simulink model "dummyModel"  (R2021a)
settings: Solver=FixedStepDiscrete  StartTime=0.0  StopTime=inf  RelTol=1e-3
libraries: simulink x1, sysauto_lib x1
settings Model: RequirementInfo="{}  %GIDa_9af0a4cd_5f44_4d95_97ed_12e2ef6ba56d"  Creator=mhochstrasser  LastModifiedBy=ge46fox
settings SolverCC: AlgebraicLoopSolver=TrustRegion  AutoInsertRateTranBlk=on
settings DataIOCC: LimitDataPoints=on  SaveOutput=off  SignalLogging=off  DSMLogging=off  SaveTime=off  ReturnWorkspaceOutputs=off
settings OptimizationCC: LifeSpan=inf
settings DebuggingCC: AlgebraicLoopMsg=error  SingleTaskRateTransMsg=error  AllowSymbolicDim=off  SFUnexpectedBacktrackingDiag=warning  SFNoUnconditionalDefaultTransitionDiag=warning  SFExecutionAtInitializationDiag=none  SFMachineParentedDataDiag=warning  ArithmeticOperatorsInVariantConditions=warning
settings SFSimCC: SimUseLocalCustomCode=off  CustomCodeUndefinedFunction=UseInterfaceOnly
settings RTWCC: RTWUseLocalCustomCode=off
settings CodeAppCC: StateflowObjectComments=on
settings GRTTargetCC: TargetLangStandard=C89/C90 (ANSI)

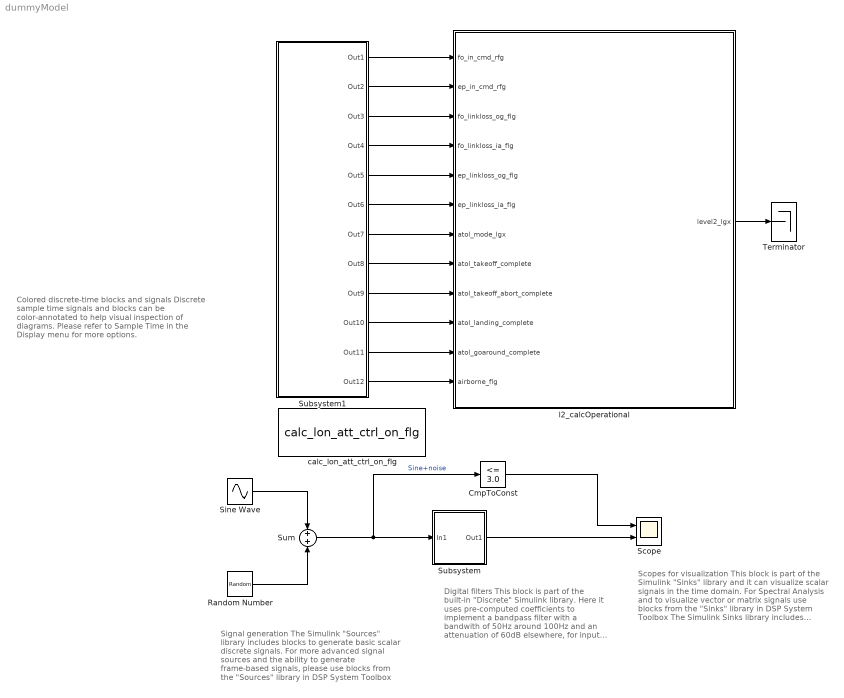
== system dummyModel ==
  note: Signal generation
      | The Simulink "Sources" library includes blocks to generate basic scalar discrete signals.
      | For more advanced signal sources and the ability to generate frame-based signals, please use blocks from the "Sources" library in DSP System Toolbox
  note: Scopes for visualization
      | This block is part of the Simulink "Sinks" library and it can visualize scalar signals in the time domain.
      | For Spectral Analysis and to visualize vector or matrix signals use blocks from the "Sinks" library in DSP System Toolbox
      |
      | The Simulink Sinks library includes scopes to visualize scalar signals in the time domain. For the Spectrum Analyzer and to viasualize vector or matrix signals refer to the Sinks library of DSP System Toolbox
  note: Digital filters
      | This block is part of the built-in "Discrete" Simulink library. Here it uses pre-computed coefficients to implement a bandpass filter with a bandwith of 50Hz around 100Hz and an attenuation of 60dB elsewhere, for input signals sampled at 8kHz.
      | To design digital filters, to select specific implementation structures, or to simulate fixed-point arithmetic use blocks from the "Filtering" library in DSP System Toolbox
  note: Colored discrete-time blocks and signals
      | Discrete sample time signals and blocks can be color-annotated to help visual inspection of diagrams. Please refer to Sample Time in the Display menu for more options.
  CmpToConst : simulink/Logic and Bit Operations/Compare To Constant  relop=<=  const=3.0  OutDataTypeStr=boolean
  Random Number : RandomNumber  RequirementInfo="{}  %GIDa_aef719ec_22fa_4968_b9f2_caf883574260"  SampleTime=1/8000
  Scope : Scope  NumInputPorts=2
  Sine Wave : Sin  Frequency=2*pi*100  Samples=1  SampleTime=1/8000
  Subsystem : Subsystem
  Subsystem1 : Subsystem
  Sum : Sum
  Terminator : Terminator
  calc_lon_att_ctrl_on_flg : sysauto_lib/calc_lon_att_ctrl_on_flg  SystemSampleTime=-1  VariantActivationTime=update diagram  Latency=0  AutoFrameSizeCalculation=off
  l2_calcOperational : Stateflow chart  TreatAsAtomicUnit=on
      settings: RTWSystemCode=Inline
  wires:
  Sum/1 -> CmpToConst/1, Subsystem/1(In1)  "Sine+noise"
  Sine Wave/1 -> Sum/1
  Random Number/1 -> Sum/2
  Subsystem/1(Out1) -> Scope/2
  CmpToConst/1 -> Scope/1
  l2_calcOperational/1(level2_lgx) -> Terminator/1
  Subsystem1/1(Out1) -> l2_calcOperational/1(fo_in_cmd_rfg)
  Subsystem1/2(Out2) -> l2_calcOperational/2(ep_in_cmd_rfg)
  Subsystem1/3(Out3) -> l2_calcOperational/3(fo_linkloss_og_flg)
  Subsystem1/4(Out4) -> l2_calcOperational/4(fo_linkloss_ia_flg)
  Subsystem1/5(Out5) -> l2_calcOperational/5(ep_linkloss_og_flg)
  Subsystem1/6(Out6) -> l2_calcOperational/6(ep_linkloss_ia_flg)
  Subsystem1/7(Out7) -> l2_calcOperational/7(atol_mode_lgx)
  Subsystem1/8(Out8) -> l2_calcOperational/8(atol_takeoff_complete)
  Subsystem1/9(Out9) -> l2_calcOperational/9(atol_takeoff_abort_complete)
  Subsystem1/10(Out10) -> l2_calcOperational/10(atol_landing_complete)
  Subsystem1/11(Out11) -> l2_calcOperational/11(atol_goaround_complete)
  Subsystem1/12(Out12) -> l2_calcOperational/12(airborne_flg)

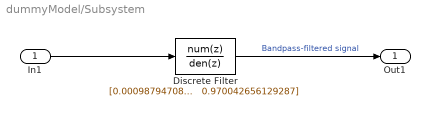
== system dummyModel/Subsystem ==
  In1 : Inport
  Discrete Filter : DiscreteFilter  RequirementInfo="{}  %GIDa_1e970cd2_fa55_4b33_ada7_a6ab44b2a5d3"  Numerator="[0.000987947087024  -0.007866111001516   0.027438142026555  -0.054764720946282   0.068409485670105  -0.054764720946282   0.027438142026555  -0.007866111001516   0.000987947087024]"  Denominator="[1.000000000000000  -7.944031997545686  27.635065757644615 -54.984635962907035  68.438574736652072 -54.568127619544200  27.217980746836638  -7.764868315600190   0.970042656129287]"
  Out1 : Outport
  wires:
  In1/1 -> Discrete Filter/1
  Discrete Filter/1 -> Out1/1  "Bandpass-filtered signal"

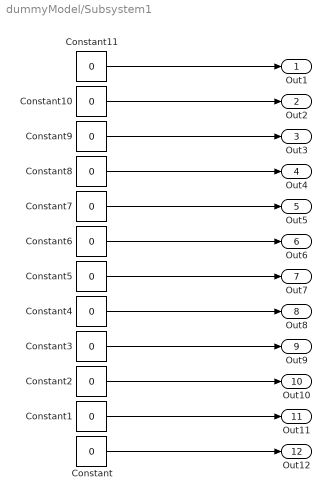
== system dummyModel/Subsystem1 ==
  Constant{,1..11} (12 alike) : Constant  Value=0  OutDataTypeStr=Inherit: Inherit via back propagation
  Out1 : Outport
  Out2 : Outport  Port=2
  Out3 : Outport  Port=3
  Out4 : Outport  Port=4
  Out5 : Outport  Port=5
  Out6 : Outport  Port=6
  Out7 : Outport  Port=7
  Out8 : Outport  Port=8
  Out9 : Outport  Port=9
  Out10 : Outport  Port=10
  Out11 : Outport  Port=11
  Out12 : Outport  Port=12
  wires:
  Constant1/1 -> Out11/1
  Constant7/1 -> Out5/1
  Constant8/1 -> Out4/1
  Constant/1 -> Out12/1
  Constant5/1 -> Out7/1
  Constant11/1 -> Out1/1
  Constant3/1 -> Out9/1
  Constant6/1 -> Out6/1
  Constant9/1 -> Out3/1
  Constant10/1 -> Out2/1
  Constant2/1 -> Out10/1
  Constant4/1 -> Out8/1

== stateflow chart dummyModel/l2_calcOperational ==
  settings: stateMachineType=MEALY_MACHINE
  state fo_in_cmd
  state ep_in_cmd
  state ep_linkloss
  state tc [group]
    state result = foincmd_folinkloss [function]
      note: /*
          | Switch from EP to FCC if either ep_linkloss or interface_error,
          | but only if the aircraft is flying, therefore a special on ground
          | link loss behaviour can be implemented
          | */
      note: /*
          |     This function is true,
          |     when ATOL prohibts automatic transition to linkloss
          | */
      (default) -> (junction 293)
      (junction 293) -> (junction 309) [order 2]
      (junction 293) -> (junction 183) [order 1] : [(((fo_linkloss_ia_flg == true)&&(airborne_flg == true))||...
          | ((fo_linkloss_og_flg == true)&&(airborne_flg == false)))]
      (junction 309) -> (junction 305) : {result = false;}
      (junction 183) -> (junction 316) [order 1] : [((atol_mode_lgx == uint8(40))&&...
          | (atol_takeoff_complete == false))||...
          | ((atol_mode_lgx == uint8(41))&&...
          | (atol_takeoff_abort_complete == false))]
      (junction 183) -> (junction 297) [order 2]
      (junction 316) -> (junction 314) : {result = false;}
      (junction 297) -> (junction 317) [order 1] : [((atol_mode_lgx == uint8(42))&&...
          | (atol_landing_complete == false))||...
          | ((atol_mode_lgx == uint8(43))&&...
          | (atol_goaround_complete == false))]
      (junction 297) -> (junction 298) [order 2] : {result = true;}
      (junction 317) -> (junction 315) : {result = false;}
      (junction 315) -> (junction 298)
      (junction 314) -> (junction 315)
      (junction 305) -> (junction 314)
    state result = x_epincmd [function]
      note: // change to EP if rising edge is detected on ep_in_cmd
      (default) -> (junction 198)
      (junction 198) -> (junction 239) [order 1] : [ep_in_cmd_rfg == true]
      (junction 198) -> (junction 197) [order 2] : {result = false;}
      (junction 239) -> (junction 240) : {result = true;}
      (junction 197) -> (junction 240)
    state result = x_foincmd [function]
      note: // change to FO if rising edge is detected on fo_in_cmd,
          | //but only if no rising edge is detected for ep_in_cmd
          | // this is needed for state ep_in_cmd transition inhibit
          | //[hasChangedTo(fao_in_cmd_flg, 1) &~ (hasChangedTo(ep_in_cmd_flg, 1))]
      (default) -> (junction 252)
      (junction 252) -> (junction 251) [order 1] : [(fo_in_cmd_rfg == true)&&...
          | (ep_in_cmd_rfg == false)]
      (junction 252) -> (junction 253) [order 2] : {result = false;}
      (junction 251) -> (junction 255) : {result = true;}
      (junction 253) -> (junction 255)
    state result = epincmd_eplinkloss [function]
      note: /*
          | Switch from EP to FCC if either ep_linkloss or interface_error,
          | but only if the aircraft is flying, therefore a special on ground
          | link loss behaviour can be implemented
          | */
      (default) -> (junction 154) : [((ep_linkloss_ia_flg == true)&&(airborne_flg == true))||...
          | ((ep_linkloss_og_flg == true)&&(airborne_flg == false))]
      (junction 154) -> (junction 156) : {result = true;}
  state ta [group]
    state foincmd_folinkloss [function]
      (default) -> (junction 134) : {level2_lgx = 2;}
    state x_epincmd [function]
      (default) -> (junction 202) : {level2_lgx = 4;}
    state x_foincmd [function]
      (default) -> (junction 212) : {level2_lgx = 5;}
    state epincmd_eplinkloss [function]
      (default) -> (junction 143) : {level2_lgx = 3;}
  state fo_linkloss
  note: ATOL is not part of this statemachine because it would lead to either (ATOL can be exited any time by any other mode commanded by fo)
      | - a inconsitent behaiviour for the fo, example: atol with no gps, he wants hlc, hlc is not possible, therefore he gets mlc (standart mode), in all other modes if he commands one mode that isn't possible he stays in the current mode
      | - many TCs that are manly used within the fo_cmd statemachine, like mode cmds, availablity
      |
      | the second possibility makes more sense but than atol is like every other mode and is therefore not avaible here but within the fo_in_cmd statemaschine
  note: © TUM-FSD, Developer: C.Krause
  fo_in_cmd -> (junction 45) [order 1] : [tc.x_epincmd() == true]
  (junction 45) -> (junction 17)
  (junction 42) -> fo_in_cmd : {ta.x_foincmd()}
  (junction 20) -> (junction 42)
  (junction 256) -> fo_in_cmd : {ta.x_foincmd()}
  fo_in_cmd -> (junction 38) [order 2] : [tc.foincmd_folinkloss() == true]
  (junction 214) -> (junction 256) [order 2] : [tc.x_foincmd() == true]
  (junction 17) -> ep_in_cmd : {ta.x_epincmd()}
  (junction 81) -> (junction 17)
  ep_in_cmd -> (junction 20) [order 1] : [tc.x_foincmd() == true]
  (junction 86) -> (junction 20)
  (junction 258) -> ep_in_cmd : {ta.x_epincmd()}
  (default) -> (junction 214)
  (junction 214) -> (junction 258) [order 1] : [tc.x_epincmd() == true]
  (junction 214) -> (junction 231) [order 3]
  ep_in_cmd -> (junction 83) [order 2] : [tc.epincmd_eplinkloss() == true]
  ep_linkloss -> (junction 86) [order 2] : [tc.x_foincmd() == true]
  (junction 91) -> (junction 86)
  (junction 231) -> (junction 83)
  (junction 83) -> ep_linkloss : {ta.epincmd_eplinkloss()}
  ep_linkloss -> (junction 81) [order 1] : [tc.x_epincmd() == true]
  (junction 88) -> (junction 81)
  fo_linkloss -> (junction 91) [order 2] : [tc.x_foincmd() == true]
  (junction 38) -> fo_linkloss : {ta.foincmd_folinkloss()}
  fo_linkloss -> (junction 88) [order 1] : [tc.x_epincmd() == true]
  data: result function_output boolean; result function_output boolean; result function_output boolean; result function_output boolean; fo_in_cmd_rfg input boolean; ep_in_cmd_rfg input boolean; fo_linkloss_og_flg input boolean; fo_linkloss_ia_flg input boolean; ep_linkloss_og_flg input boolean; ep_linkloss_ia_flg input boolean; level2_lgx output int32; atol_mode_lgx input uint8; atol_takeoff_complete input boolean; atol_takeoff_abort_complete input; atol_landing_complete input boolean; atol_goaround_complete input; airborne_flg input boolean
